simulink model "PI_controller_alpha1"  (R2019b)
settings: Solver=FixedStepAuto  StartTime=0.0  StopTime=30  FixedStep=0.005  RelTol=1e-3
settings Model: Creator=suvo  LastModifiedBy=suvo

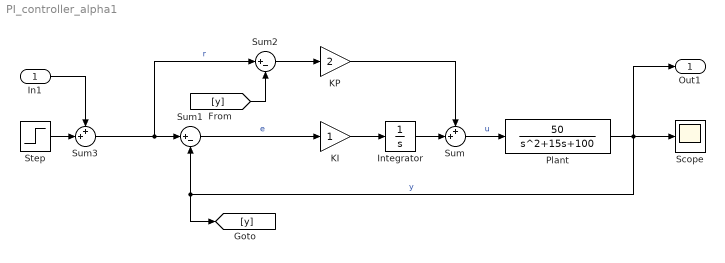
== system PI_controller_alpha1 ==
  In1 : Inport
  Integrator : Integrator
  KI : Gain
  KP : Gain  Gain=2
  Plant : TransferFcn  Numerator=50  Denominator=[1 15 100]
  Scope : Scope
  Step : Step  SampleTime=0
  Sum : Sum  Inputs=++|
  Sum1 : Sum  Inputs=|+-
  Sum2 : Sum  Inputs=|+-
  Sum3 : Sum  Inputs=++|
  Out1 : Outport
  wires:
  KI/1 -> Integrator/1
  Sum1/1 -> KI/1  "e"
  Plant/1 -> Scope/1, Out1/1, [y], Sum1/2  "y"
  Sum3/1 -> Sum2/1, Sum1/1  "r"
  Sum2/1 -> KP/1
  KP/1 -> Sum/1
  Integrator/1 -> Sum/2
  Sum/1 -> Plant/1  "u"
  In1/1 -> Sum3/1
  Step/1 -> Sum3/2
  [y] -> Sum2/2
